simulink model "Lab_Electromechanical_System"  (R2018a)
settings: Solver=VariableStepAuto  StartTime=0.0  StopTime=3e-3  RelTol=1e-3
libraries: dspsrcs4 x1
settings Model: Creator=samak-twins  LastModifiedBy=samak

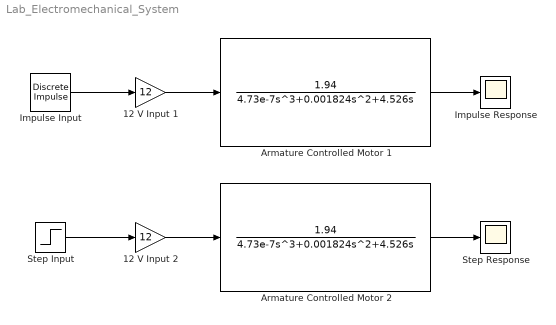
== system Lab_Electromechanical_System ==
  12 V Input 1 : Gain  Gain=12
  12 V Input 2 : Gain  Gain=12
  Armature Controlled Motor 1 : TransferFcn  Numerator=[1.94]  Denominator=[4.73e-7 0.001824 4.526 0]
  Armature Controlled Motor 2 : TransferFcn  Numerator=[1.94]  Denominator=[4.73e-7 0.001824 4.526 0]
  Impulse Input : dspsrcs4/Discrete  Impulse  Delay=0  SampleTime=0.0001  FrameSample=1  OutputFrames=off  dataType=double  isSigned=on  wordLen=16  udDataType=sfix(16)  fracBitsMode=Best precision  numFracBits=15  OutDataTypeStr=double  LastOutDataTypeStr=double
  Impulse Response : Scope
  Step Input : Step  Time=0  SampleTime=0
  Step Response : Scope
  wires:
  Armature Controlled Motor 2/1 -> Step Response/1
  Step Input/1 -> 12 V Input 2/1
  Armature Controlled Motor 1/1 -> Impulse Response/1
  Impulse Input/1 -> 12 V Input 1/1
  12 V Input 1/1 -> Armature Controlled Motor 1/1
  12 V Input 2/1 -> Armature Controlled Motor 2/1
